simulink model "fuzzy_rocky_optimized"  (R2021a)
settings: Solver=VariableStepAuto  StartTime=0.0  StopTime=45.0  RelTol=1e-3
undefined symbols (not defined in the file or in its folder): sigbuilder_block
libraries: fuzblock x1
settings Model: Creator=blan  LastModifiedBy=blan

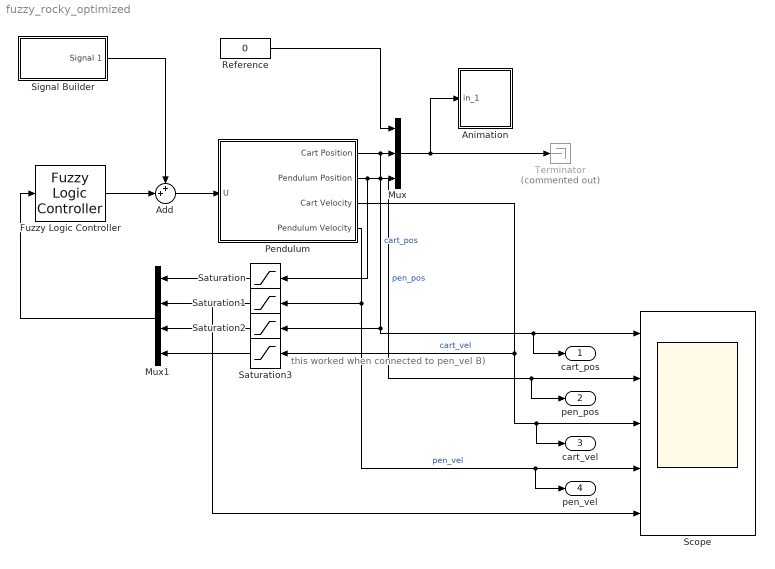
== system fuzzy_rocky_optimized ==
  note: this worked when connected to pen_vel B)
  Add : Sum  Inputs=++|
  Animation : Subsystem  mask(Pendulum plot){RefBlock=Reference}
      mask prompts: RefBlock "DC reference signal block name:"
      mask help: Pendulum plot
      mask Help: Pendulum animation function using Handle graphics.
      mask Display: plot([-10 10],[0 0],[-2 -2 2 2],[0 1 1 0],[0 3],[1 5])
  Fuzzy Logic Controller : fuzblock/Fuzzy Logic  Controller  FIS=fisMFTuned  OutputSampleNumber=101  DataType=double  FuzzifiedInputs=off  RuleFiringStrengths=off  RuleOutputs=off  AggregatedOutputs=off  SimulateUsing=Interpreted execution  OutOfRangeInputValueMessage=warning  NoRuleFiredMessage=warning  EmptyOutputFuzzySetMessage=warning
  Mux : Mux  Inputs=3
  Mux1 : Mux
  Pendulum : Subsystem  mask(Inverted pendulum on cart){Mcart=0.455, m=0.21, l=0.61/2, g=9.8}
      mask prompts: Mcart "Mass of cart (kg):"; m "Mass of pendulum (kg):"; l "Distance to pendulum center of mass(m):"; g "Acceleration of gravity (m/s^2):"
      mask help: Unmask and double-click to see dynamics
      mask Help: Nonlinear dynamics of inverted pendulum on cart.
  Reference : Constant  Value=0
  Saturation : Saturate  UpperLimit=pi  LowerLimit=-pi
  Saturation1 : Saturate  UpperLimit=5  LowerLimit=-5
  Saturation2 : Saturate  UpperLimit=10  LowerLimit=-10
  Saturation3 : Saturate  UpperLimit=5  LowerLimit=-5
  Scope : Scope  NumInputPorts=5
  Signal Builder : Subsystem  Tag=STV Subsys  LoadFcn=sigbuilder_block('load');  StartFcn=sigbuilder_block('start');  StopFcn=sigbuilder_block('stop');  ClipboardFcn=sigbuilder_block('clipboard');  mask(Sigbuilder block){tuvar=[0:10]}
      mask help: Simulink:masks:SigbuilderBlock_MD
      mask init:
      | if ~strcmp(get_param(bdroot(gcbh),'SimulationStatus'),'stopped') tuvar = sigbuilder_block('maskInit'); end
      settings: CopyFcn=sigbuilder_block('copy');  DeleteFcn=sigbuilder_block('delete');  ModelCloseFcn=sigbuilder_block('modelClose');  PreSaveFcn=sigbuilder_block('preSave');  PauseFcn=sigbuilder_block('pause');  ContinueFcn=sigbuilder_block('continue');  NameChangeFcn=sigbuilder_block('namechange');  OpenFcn=sigbuilder_block('open',[352.5 85 550.5 362.5 ]);  CloseFcn=sigbuilder_block('close');
      mask Display: plot(0, 0, 100, 100,[2, 2, 32, 32, 2], [68, 8, 8, 68, 68],[32, 2], [38, 38], [32, 19, 2],[53, 60, 44], [32, 17, 17, 2],[16, 16, 31, 31]);txt = getActiveGroup(gcbh);text(2, 100, txt,'verticalAlignment', 'top');
  Terminator : Terminator  Commented=on
  cart_pos : Outport  OutDataTypeStr=double
  pen_pos : Outport  Port=2  OutDataTypeStr=double
  cart_vel : Outport  Port=3  OutDataTypeStr=double
  pen_vel : Outport  Port=4  OutDataTypeStr=double
  wires:
  Pendulum/1(Cart Position) -> cart_pos/1, Scope/1, Saturation2/1, Mux/2  "cart_pos"
  Pendulum/2(Pendulum Position) -> Saturation/1, pen_pos/1, Scope/2, Mux/3  "pen_pos"
  Reference/1 -> Mux/1
  Fuzzy Logic Controller/1 -> Add/2
  Signal Builder/1(Signal 1) -> Add/1
  Add/1 -> Pendulum/1(U)
  Pendulum/4(Pendulum Velocity) -> pen_vel/1, Scope/4, Saturation1/1  "pen_vel"
  Mux1/1 -> Fuzzy Logic Controller/1
  Pendulum/3(Cart Velocity) -> cart_vel/1, Scope/3, Saturation3/1  "cart_vel"
  Mux/1 -> Terminator/1, Animation/1(in_1)
  Saturation/1 -> Mux1/1
  Saturation1/1 -> Scope/5, Mux1/2
  Saturation2/1 -> Mux1/3
  Saturation3/1 -> Mux1/4

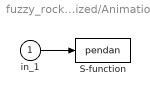
== system fuzzy_rocky_optimized/Animation ==
  in_1 : Inport
  S-function : S-Function  FunctionName=pendan  Parameters=RefBlock  SFunctionDeploymentMode=off  EnableBusSupport=off
      settings: DeleteFcn=pendan([],[],[],'DeleteBlock');
  wires:
  in_1/1 -> S-function/1

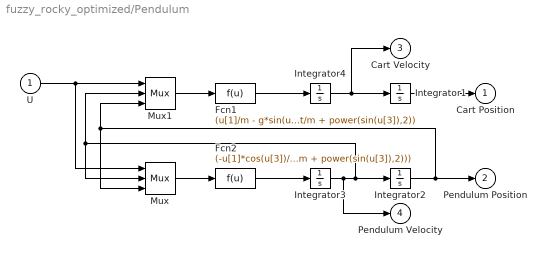
== system fuzzy_rocky_optimized/Pendulum ==
  U : Inport
  Fcn1 : Fcn  Expr=(u[1]/m - g*sin(u[3])*cos(u[3]) + l*power(u[2],2)*sin(u[3]))/(Mcart/m + power(sin(u[3]),2))
  Fcn2 : Fcn  Expr=(-u[1]*cos(u[3])/m + (Mcart+m)*g*sin(u[3])/m - l*power(u[2],2)*sin(u[3])*cos(u[3]))/(l*(Mcart/m + power(sin(u[3]),2)))
  Integrator{1..4} (4 alike) : Integrator
  Mux : Mux  Inputs=3
  Mux1 : Mux  Inputs=3
  Cart Position : Outport  InitialOutput=0  VectorParamsAs1DForOutWhenUnconnected=off
  Pendulum Position : Outport  Port=2  InitialOutput=0  VectorParamsAs1DForOutWhenUnconnected=off
  Cart Velocity : Outport  Port=3  InitialOutput=0  VectorParamsAs1DForOutWhenUnconnected=off
  Pendulum Velocity : Outport  Port=4  InitialOutput=0  VectorParamsAs1DForOutWhenUnconnected=off
  wires:
  Integrator1/1 -> Cart Position/1
  Fcn2/1 -> Integrator3/1
  Mux/1 -> Fcn2/1
  Mux1/1 -> Fcn1/1
  Fcn1/1 -> Integrator4/1
  Integrator4/1 -> Cart Velocity/1, Integrator1/1
  U/1 -> Mux1/1, Mux/1
  Integrator3/1 -> Pendulum Velocity/1, Integrator2/1, Mux1/2, Mux/2
  Integrator2/1 -> Pendulum Position/1, Mux1/3, Mux/3

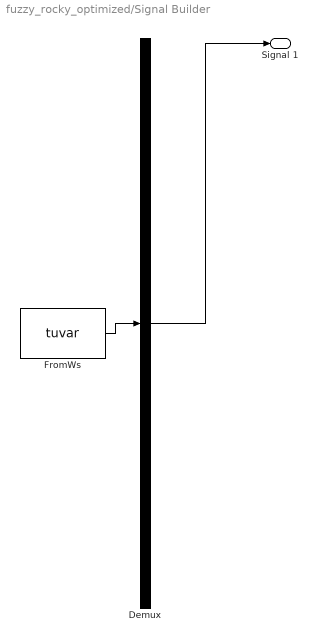
== system fuzzy_rocky_optimized/Signal Builder ==
  Demux : Demux  Tag=STV Demux  Outputs=1
      settings: DisplayOption=none
  FromWs : FromWorkspace  Tag=STV FromWs  VariableName=tuvar
      SigBuilderData=|
      | common.afterFinalStr = 'Extrapolate'
      | common.sampleTime = 0
      | dataSet.timeRange = [0 10]
      | dataSet.name = 'Group 1'
      | sbobj.Groups.Name = 'Group 1'
      | sbobj.Groups.Signals.Name = 'Signal 1'
      | sbobj.Groups.Signals.XData = [0 4.84 4.84 5 5 10]
      | sbobj.Groups.Signals.YData = [0 0 8 8 0 0]
  Signal 1 : Outport  Tag=STV Outport
  wires:
  Demux/1 -> Signal 1/1
  FromWs/1 -> Demux/1
